simulink model "sample_road_profile_model"  (R2026a)
settings: Solver=VariableStepAuto  StopTime=20
libraries: nesl_utility x2, fl_lib x1
settings Model: Creator=isaacito  LastModifiedBy=isaacito

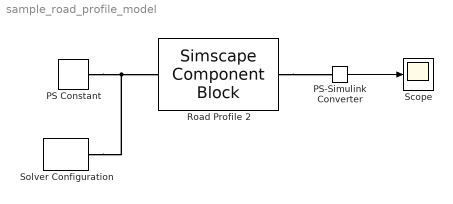
== system sample_road_profile_model ==
  PS Constant : fl_lib/Physical Signals/Sources/PS Constant  constant=0.8 m/s
  PS-Simulink Converter : nesl_utility/PS-Simulink Converter  PhysicalDomain=network_engine_domain  SubClassName=ps_output  LeftPortType=input  RightPortType=output  PseudoPeriodic=off  Frequencies=[]  VectorFormat=inherit  Unit=deg  AffineConversion=off
  Road Profile 2 : SimscapeComponentBlock  SourceFile=SimpleRoadProfile2  ComponentPath=SimpleRoadProfile2  ComponentVariants="[\"SimpleRoadProfile2\"]"  ComponentVariantNames="[\"SimpleRoadProfile2\"]"  ClassName=SimpleRoadProfile2  SchemaVersion=1  x_vector=[-10, -2, -1, 0, 1, 10, 11, 12, 20] m  angle_vector=[0, 0, 0, 5, 5, 5, 0, 0, 0] deg  profile_interp_method=simscape.enum.interpolation.smooth  x_specify=on  x_priority=High  x=-2 m  x_nominal_specify=off  x_nominal_value=1  x_nominal_unit=m
      settings: CopyFcn=simscape.sscblock.internal.componentBlockCallback(gcbh,'COPY')  PreCopyFcn=simscape.sscblock.internal.componentBlockCallback(gcbh,'PRECOPY')  PreDeleteFcn=simscape.sscblock.internal.componentBlockCallback(gcbh,'PREDELETE')
      mask Type: Simple Road Profile
  Scope : Scope
      settings: ActiveDisplayYMinimum=-0.625  ActiveDisplayYMaximum=5.6250000000000009
  Solver Configuration : nesl_utility/Solver Configuration  PhysicalDomain=network_engine_domain  SubClassName=solver  LeftPortType=input  RightPortType=generic  Tones=[]  Harmonics=[]  SimulateNoise=off  Profile=off  UseLocalSampling=off  EnableSwitchedLinearOptims=on  FrequencyDomain=off  UseCCode=off  RelTol=0.001  AbsTol=0.001  MinStep=1e-09  ToWorkspace=off  RevertToSquareIcSolve=off  NumHomotopyIterations=100  PhasorMode=off  PhasorModeNumHarmonics=1  ConsistencySolver=NEWTON_XTOL_AFTER_FTOL  CanonicalOrdering=CANONICAL  OptimizeIntermediates=OPTIMIZED  IndexReductionMethod=DerivativeReplacement  DoDC=off  ResidualTolerance=1e-09  ConsistencyTolSource=GLOBAL  ConsistencyAbsTol=0.001  ConsistencyRelTol=0.001  ConsistencyTolFactor=0.001  UseLocalSolver=off  LocalSolverChoice=NE_BACKWARD_EULER_ADVANCER  ResolveIndetEquations=on  FunctionEvalNumThread=1  LocalSolverSampleTime=0.001  DoFixedCost=off  MaxNonlinIter=3  MaxModeIter=2  ComputeImpulses=off  ImpulseIterations=2  LinearAlgebra=auto  LinearAlgebraNumThread=0  EquationFormulation=NE_TIME_EF  DelaysMemoryBudget=1024  AutomaticFiltering=on  FilteringTimeConstant=0.001  PartitionStorageMethod=AS_NEEDED  PartitionMemoryBudget=1024  PartitionMethod=ROBUST  MultibodyUseLocalSolver=off  MultibodyLocalSolverChoice=ODE1  MultibodyLocalSolverSampleTime=0.001
  wires:
  PS-Simulink Converter/1 -> Scope/1
  connections:
  PS Constant/RConn1 -- Solver Configuration/RConn1 -- Road Profile 2/LConn1
  Road Profile 2/RConn1 -- PS-Simulink Converter/LConn1
